simulink model "VOO_Pacemaker"  (R2020a)
settings: Solver=FixedStepAuto  StartTime=0.0  StopTime=10.0  FixedStep=1e-3  RelTol=1e-3  EnableMultiTasking=on
settings Model: ExtModeTrigDuration=5  Creator=vinee  LastModifiedBy=Mitch
settings OptimizationCC: EnhancedBackFolding=on  PassReuseOutputArgsAs=Individual arguments  ZeroExternalMemoryAtStartup=off  ZeroInternalMemoryAtStartup=off  MaxStackSize=64  OptimizeBlockOrder=speed  DifferentSizesBufferReuse=on  OptimizationCustomize=off  EfficientTunableParamExpr=on
settings DebuggingCC: ParameterTunabilityLossMsg=error
settings HardwareCC: ProdBitPerPointer=32  ProdBitPerSizeT=32  ProdBitPerPtrDiffT=32  ProdLargestAtomicInteger=Long  ProdLargestAtomicFloat=Double  ProdWordSize=32  ProdHWDeviceType=ARM Compatible->ARM Cortex
settings SFSimCC: MATLABDynamicMemAlloc=off
settings RTWCC: SystemTargetFile=ert.tlc  HardwareBoard=NXP FRDM-K64F  TemplateMakefile=ert_default_tmf  Toolchain=GNU Tools for ARM Embedded Processors
settings CodeAppCC: ForceParamTrailComments=on  IgnoreCustomStorageClasses=off  OperatorAnnotations=on  SimulinkDataObjDesc=on  SFDataObjDesc=on  InsertBlockDesc=on

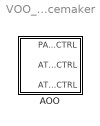
== system VOO_Pacemaker ==
  AOO : Stateflow chart  TreatAsAtomicUnit=on

== stateflow chart VOO_Pacemaker/AOO ==
  state VOO
    entry:
    Z_ATR_CTRL = 0;
    Z_VENT_CTRL =0;
    ATR_GND_CTRL = 0;
    ATR_PACE_CTRL =0;
    PACE_GND_CTRL = 1;
    PACING_REF_PWM = BLANK;
    state DISCHARGE_C22
      entry:
      PACE_CHARGE_CTRL = 0;
      VENT_PACE_CTRL = 1;
      VENT_GND_CTRL = 0;
    state CHARGE_C22
      entry:
      VENT_PACE_CTRL = 0;
      VENT_GND_CTRL = 1;
      PACE_CHARGE_CTRL =1;
    (default) -> VOO.CHARGE_C22
    VOO.DISCHARGE_C22 -> VOO.CHARGE_C22 : [after(VPWM ,msec)]
    VOO.CHARGE_C22 -> VOO.DISCHARGE_C22 : [after(VPWM, msec)]
  state VVI
    entry:
    Z_ATR_CTRL = 0;
    Z_VENT_CTRL =0;
    ATR_GND_CTRL = 0;
    ATR_PACE_CTRL =0;
    PACE_GND_CTRL = 1;
    PACING_REF_PWM = BLANK;
    state DISCHARGE_C22
      entry:
      PACE_CHARGE_CTRL = 0;
      VENT_PACE_CTRL = 1;
      VENT_GND_CTRL = 0;
    note: after(VPWM ,msec)
    state CHARGE_C22
      entry:
      VENT_PACE_CTRL = 0;
      VENT_GND_CTRL = 1;
      PACE_CHARGE_CTRL =1;
    note: after(VPWM, msec)
    state ?
    (default) -> VVI.CHARGE_C22
    VVI.DISCHARGE_C22 -> VVI.CHARGE_C22
    VVI.CHARGE_C22 -> VVI.DISCHARGE_C22
    VVI -> VVI
  data: PACE_CHARGE_CTRL output; ATR_GND_CTRL output; ATR_PACE_CTRL output
